simulink model "Exemplu1_pag2_cazul_I"  (R2021b)
settings: Solver=VariableStepAuto  StartTime=0.0  StopTime=300  RelTol=1e-6
settings Model: Creator=alexandra.szedlak-st  LastModifiedBy=alexandra.szedlak-st

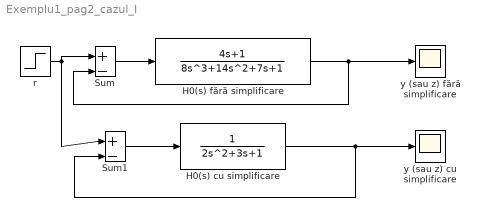
== system Exemplu1_pag2_cazul_I ==
  H0(s) cu simplificare : TransferFcn  Denominator=[2 3 1]
  H0(s) fără simplificare : TransferFcn  Numerator=[4 1]  Denominator=[8 14 7 1]
  Sum : Sum  Inputs=|+-
  Sum1 : Sum  Inputs=|+-
  r : Step  Time=0  After=10  SampleTime=0
  y (sau z) cu simplificare : Scope
  y (sau z) fără simplificare : Scope
  wires:
  H0(s) fără simplificare/1 -> Sum/2, y (sau z) fără simplificare/1
  H0(s) cu simplificare/1 -> Sum1/2, y (sau z) cu simplificare/1
  Sum/1 -> H0(s) fără simplificare/1
  r/1 -> Sum1/1, Sum/1
  Sum1/1 -> H0(s) cu simplificare/1
